simulink library "INT_Rail_CtlLoopLimMeUn"  (R2016b)
settings: Solver=VariableStepAuto  StartTime=0.0  StopTime=10.0  RelTol=1e-3
settings Model: Creator=Administrator  LastModifiedBy=Administrator

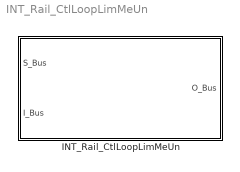
== system INT_Rail_CtlLoopLimMeUn ==
  INT_Rail_CtlLoopLimMeUn : Subsystem

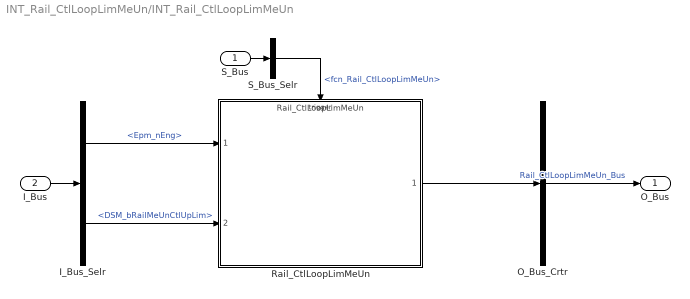
== system INT_Rail_CtlLoopLimMeUn/INT_Rail_CtlLoopLimMeUn ==
  S_Bus : Inport
  I_Bus : Inport  Port=2
  I_Bus_Selr : BusSelector  OutputSignals=Epm_nEng,DSM_bRailMeUnCtlUpLim
  O_Bus_Crtr : BusCreator  Inputs=1
  Rail_CtlLoopLimMeUn : ModelReference  ModelNameDialog=Rail_CtlLoopLimMeUn  SimulationMode=Normal  ModelReferenceVersion=1.4  TriggerPortName=function  TriggerPortTriggerType=function-call  TriggerPortStatesWhenEnabling=held
  S_Bus_Selr : BusSelector  OutputSignals=fcn_Rail_CtlLoopLimMeUn
  O_Bus : Outport
  wires:
  S_Bus_Selr/1 -> Rail_CtlLoopLimMeUn/Trigger  "<fcn_Rail_CtlLoopLimMeUn>"
  S_Bus/1 -> S_Bus_Selr/1
  I_Bus/1 -> I_Bus_Selr/1
  I_Bus_Selr/1 -> Rail_CtlLoopLimMeUn/1  "<Epm_nEng>"
  I_Bus_Selr/2 -> Rail_CtlLoopLimMeUn/2  "<DSM_bRailMeUnCtlUpLim>"
  O_Bus_Crtr/1 -> O_Bus/1  "Rail_CtlLoopLimMeUn_Bus"
  Rail_CtlLoopLimMeUn/1 -> O_Bus_Crtr/1
